simulink library "QuadratureEncoder"  (R2022b)
settings: Solver=VariableStepAuto  StartTime=0.0  StopTime=10.0  RelTol=1e-3
libraries: simulink x1
settings Model: Creator=vallabhad  LastModifiedBy=vallabhad

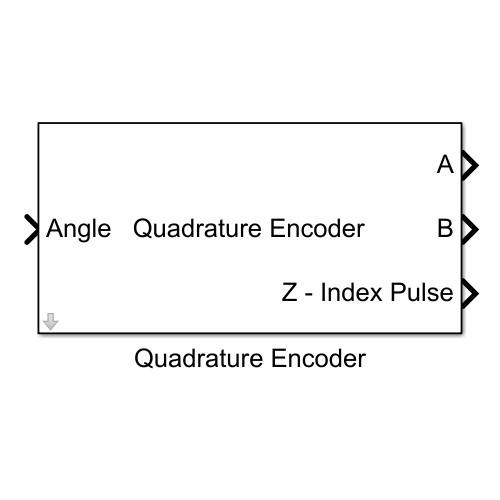
[thumbnail: Simulink's stored preview of the top-level diagram]
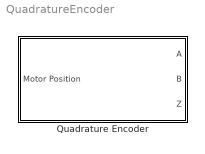
== system QuadratureEncoder ==
  Quadrature Encoder : Subsystem  mask(Quadrature Encoder){PPR=1024}
      mask prompts: PPR "PPR (Pulses Per Revolution)"
      mask help: A simple quadrature encoder that generates A, B & Z pulses that can be used to find the poistion and speed of a motor.
      mask DialogControl DescGroupVar Prompt: Quadrature Encoder
      mask DialogControl DescTextVar Prompt: Generates A, B & Z pulses depending on the motor position
      mask DialogControl Control3 Prompt: An Index pulse will be generated after no. of pulses specifed in the PPR
      mask DialogControl Control5 Prompt: Reference Paper link :
      mask DialogControl Control4 Prompt: https://real-j.mtak.hu/24586/1/Acta_Electrical_2010_2.pdf#page=29
      mask Display:
      | disp('Quadrature Encoder');
      | port_label('input', 1, ['Angle']);
      | port_label('output', 1, 'A');
      | port_label('output', 2, 'B');
      | port_label('output', 3, 'Z - Index Pulse');

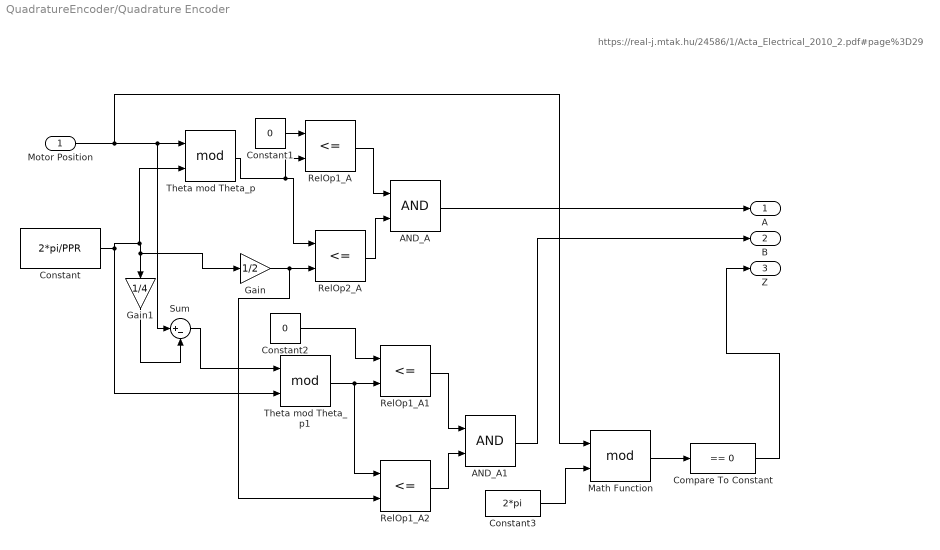
== system QuadratureEncoder/Quadrature Encoder ==
  note: https://real-j.mtak.hu/24586/1/Acta_Electrical_2010_2.pdf#page%3D29
  Motor Position : Inport
  AND_A : Logic  AllPortsSameDT=off  OutDataTypeStr=boolean
  AND_A1 : Logic  AllPortsSameDT=off  OutDataTypeStr=boolean
  Compare To Constant : simulink/Logic and Bit Operations/Compare To Constant  relop===  const=0  OutDataTypeStr=boolean
  Constant : Constant  Value=2*pi/PPR  SampleTime=-1
  Constant1 : Constant  Value=0  SampleTime=-1
  Constant2 : Constant  Value=0  SampleTime=-1
  Constant3 : Constant  Value=2*pi  SampleTime=-1
  Gain : Gain  Gain=1/2
  Gain1 : Gain  Gain=1/4
  Math Function : Math  Operator=mod
  RelOp1_A : RelationalOperator  Operator=<=  OutDataTypeStr=boolean  RndMeth=Simplest  InputSameDT=off
  RelOp1_A1 : RelationalOperator  Operator=<=  OutDataTypeStr=boolean  RndMeth=Simplest  InputSameDT=off
  RelOp1_A2 : RelationalOperator  Operator=<=  OutDataTypeStr=boolean  RndMeth=Simplest  InputSameDT=off
  RelOp2_A : RelationalOperator  Operator=<=  OutDataTypeStr=boolean  RndMeth=Simplest  InputSameDT=off
  Sum : Sum  Inputs=|+-
  Theta mod Theta_p : Math  Operator=mod
  Theta mod Theta_p1 : Math  Operator=mod
  A : Outport
  B : Outport  Port=2
  Z : Outport  Port=3
  wires:
  Compare To Constant/1 -> Z/1
  RelOp1_A2/1 -> AND_A1/2
  AND_A1/1 -> B/1
  Theta mod Theta_p1/1 -> RelOp1_A2/1, RelOp1_A1/2
  Constant1/1 -> RelOp1_A/1
  Gain/1 -> RelOp1_A2/2, RelOp2_A/2
  Math Function/1 -> Compare To Constant/1
  Motor Position/1 -> Math Function/1, Sum/1, Theta mod Theta_p/1
  RelOp2_A/1 -> AND_A/2
  AND_A/1 -> A/1
  Theta mod Theta_p/1 -> RelOp2_A/1, RelOp1_A/2
  RelOp1_A1/1 -> AND_A1/1
  Constant/1 -> Theta mod Theta_p/2, Gain1/1, Gain/1, Theta mod Theta_p1/2
  Constant2/1 -> RelOp1_A1/1
  Sum/1 -> Theta mod Theta_p1/1
  Constant3/1 -> Math Function/2
  Gain1/1 -> Sum/2
  RelOp1_A/1 -> AND_A/1
